simulink model "sim_BTMS"  (R2018b)
settings: Solver=FixedStepAuto  StartTime=0.0  StopTime=SimPara.t_sim  FixedStep=SimPara.t_step  RelTol=1e-3
values from neighbouring files (symbols this model uses):
  p = epe(jj).p    [main_sim_BTMS.m]    (also in main_sim_BTMS_1_system_setup.m = epe_mod(jj).p)
  SysPara = rmfield(SysPara, {'p','s'})    [main_sim_BTMS_1_system_setup.m]
undefined symbols (not defined in the file or in its folder): A, BatPara, BTMSConfig, i, LSAPara, SimPara, x2_cal, x3_cal, x_cal
libraries: simulink x14, dspstat3 x7, dspindex x1
(part 2 of 4)

== system sim_BTMS/Battery system simulation/Static and dynamic LIB parameters/LIB Parameter Look-Ups ==
  note: Determination of the current BatPara cell parameter set, dependent on SOC, C-Rate and Temperature of every individual cell of the battery system.
  note: RC-Element 1
  note: RC-Element 2
  note: RC-Element 3
  note: RC-Element 4
  BatState_th_in : Inport
  BatState_el_in : Inport  Port=2
  Apply Deviation Map to C_A : Constant  Value=BatPara.electrical.C_A*SysPara.DeviationMap.C_A  VectorParams1D=off
  Bus Creator : BusCreator  Inputs=10
  Bus Selector : BusSelector  OutputSignals=SOC,I_cell [A]
  Bus Selector1 : BusSelector  OutputSignals=T_cell [°C]
  Divide : Product  Inputs=*/
  Lookup C1 : Lookup_n-D  NumberOfTableDimensions=3  BreakpointsForDimension1=BatPara.electrical.dyn.SOC  BreakpointsForDimension2=BatPara.electrical.dyn.T  BreakpointsForDimension3=BatPara.electrical.dyn.C_rate  BeginIndexSearchUsingPreviousIndexResult=on  Table=BatPara.electrical.dyn.C1  ExtrapMethod=Clip  RemoveProtectionInput=on  UseLastTableValue=on  InternalRulePriority=Speed  RndMeth=Simplest  InputSameDT=on
  Lookup C2 : Lookup_n-D  NumberOfTableDimensions=3  BreakpointsForDimension1=BatPara.electrical.dyn.SOC  BreakpointsForDimension2=BatPara.electrical.dyn.T  BreakpointsForDimension3=BatPara.electrical.dyn.C_rate  BeginIndexSearchUsingPreviousIndexResult=on  Table=BatPara.electrical.dyn.C2  ExtrapMethod=Clip  RemoveProtectionInput=on  UseLastTableValue=on  InternalRulePriority=Speed  RndMeth=Simplest  InputSameDT=on
  Lookup C3 : Lookup_n-D  NumberOfTableDimensions=3  BreakpointsForDimension1=BatPara.electrical.dyn.SOC  BreakpointsForDimension2=BatPara.electrical.dyn.T  BreakpointsForDimension3=BatPara.electrical.dyn.C_rate  BeginIndexSearchUsingPreviousIndexResult=on  Table=BatPara.electrical.dyn.C3  ExtrapMethod=Clip  RemoveProtectionInput=on  UseLastTableValue=on  InternalRulePriority=Speed  RndMeth=Simplest  InputSameDT=on
  Lookup C4 : Lookup_n-D  NumberOfTableDimensions=3  BreakpointsForDimension1=BatPara.electrical.dyn.SOC  BreakpointsForDimension2=BatPara.electrical.dyn.T  BreakpointsForDimension3=BatPara.electrical.dyn.C_rate  BeginIndexSearchUsingPreviousIndexResult=on  Table=BatPara.electrical.dyn.C4  ExtrapMethod=Clip  RemoveProtectionInput=on  UseLastTableValue=on  InternalRulePriority=Speed  RndMeth=Simplest  InputSameDT=on
  Lookup R1 : Lookup_n-D  NumberOfTableDimensions=3  BreakpointsForDimension1=BatPara.electrical.dyn.SOC  BreakpointsForDimension2=BatPara.electrical.dyn.T  BreakpointsForDimension3=BatPara.electrical.dyn.C_rate  BeginIndexSearchUsingPreviousIndexResult=on  Table=BatPara.electrical.dyn.R1  ExtrapMethod=Clip  RemoveProtectionInput=on  UseLastTableValue=on  InternalRulePriority=Speed  RndMeth=Simplest  InputSameDT=on
  Lookup R2 : Lookup_n-D  NumberOfTableDimensions=3  BreakpointsForDimension1=BatPara.electrical.dyn.SOC  BreakpointsForDimension2=BatPara.electrical.dyn.T  BreakpointsForDimension3=BatPara.electrical.dyn.C_rate  BeginIndexSearchUsingPreviousIndexResult=on  Table=BatPara.electrical.dyn.R2  ExtrapMethod=Clip  RemoveProtectionInput=on  UseLastTableValue=on  InternalRulePriority=Speed  RndMeth=Simplest  InputSameDT=on
  Lookup R3 : Lookup_n-D  NumberOfTableDimensions=3  BreakpointsForDimension1=BatPara.electrical.dyn.SOC  BreakpointsForDimension2=BatPara.electrical.dyn.T  BreakpointsForDimension3=BatPara.electrical.dyn.C_rate  BeginIndexSearchUsingPreviousIndexResult=on  Table=BatPara.electrical.dyn.R3  ExtrapMethod=Clip  RemoveProtectionInput=on  UseLastTableValue=on  InternalRulePriority=Speed  RndMeth=Simplest  InputSameDT=on
  Lookup R4 : Lookup_n-D  NumberOfTableDimensions=3  BreakpointsForDimension1=BatPara.electrical.dyn.SOC  BreakpointsForDimension2=BatPara.electrical.dyn.T  BreakpointsForDimension3=BatPara.electrical.dyn.C_rate  BeginIndexSearchUsingPreviousIndexResult=on  Table=BatPara.electrical.dyn.R4  ExtrapMethod=Clip  RemoveProtectionInput=on  UseLastTableValue=on  InternalRulePriority=Speed  RndMeth=Simplest  InputSameDT=on
  Lookup R_0 : Lookup_n-D  NumberOfTableDimensions=3  BreakpointsForDimension1=BatPara.electrical.dyn.SOC  BreakpointsForDimension2=BatPara.electrical.dyn.T  BreakpointsForDimension3=BatPara.electrical.dyn.C_rate  BeginIndexSearchUsingPreviousIndexResult=on  Table=BatPara.electrical.dyn.R_0  ExtrapMethod=Clip  RemoveProtectionInput=on  UseLastTableValue=on  InternalRulePriority=Speed  RndMeth=Simplest  InputSameDT=on
  BatPara_el_uniform : Outport
  wires:
  Bus Selector/1 -> Lookup R_0/1, Lookup R1/1, Lookup C1/1, Lookup C4/1, Lookup R4/1, Lookup C3/1, Lookup R3/1, Lookup C2/1, Lookup R2/1  "<SOC>"
  Divide/1 -> Lookup R_0/2, Lookup R1/2, Lookup C1/2, Lookup C4/2, Lookup R4/2, Lookup C3/2, Lookup R3/2, Lookup C2/2, Lookup R2/2
  Lookup R_0/1 -> Bus Creator/1  "R_0 [Ohm]"
  Bus Selector1/1 -> Lookup R3/3, Lookup C3/3, Lookup R4/3, Lookup C4/3, Lookup R_0/3, Lookup R1/3, Lookup C1/3, Lookup R2/3, Lookup C2/3  "<T_cell [°C]>"
  Lookup R1/1 -> Bus Creator/2  "R1 [Ohm]"
  Lookup R2/1 -> Bus Creator/4  "R2 [Ohm]"
  Lookup C1/1 -> Bus Creator/3  "C1 [F]"
  Lookup C2/1 -> Bus Creator/5  "C2 [F]"
  BatState_el_in/1 -> Bus Selector/1
  Apply Deviation Map to C_A/1 -> Divide/2, Bus Creator/10  "C_A [Ah]"
  Bus Creator/1 -> BatPara_el_uniform/1
  Bus Selector/2 -> Divide/1  "<I_cell [A]>"
  BatState_th_in/1 -> Bus Selector1/1
  Lookup C4/1 -> Bus Creator/9  "C4 [F]"
  Lookup C3/1 -> Bus Creator/7  "C3 [F]"
  Lookup R4/1 -> Bus Creator/8  "R4 [Ohm]"
  Lookup R3/1 -> Bus Creator/6  "R3 [Ohm]"

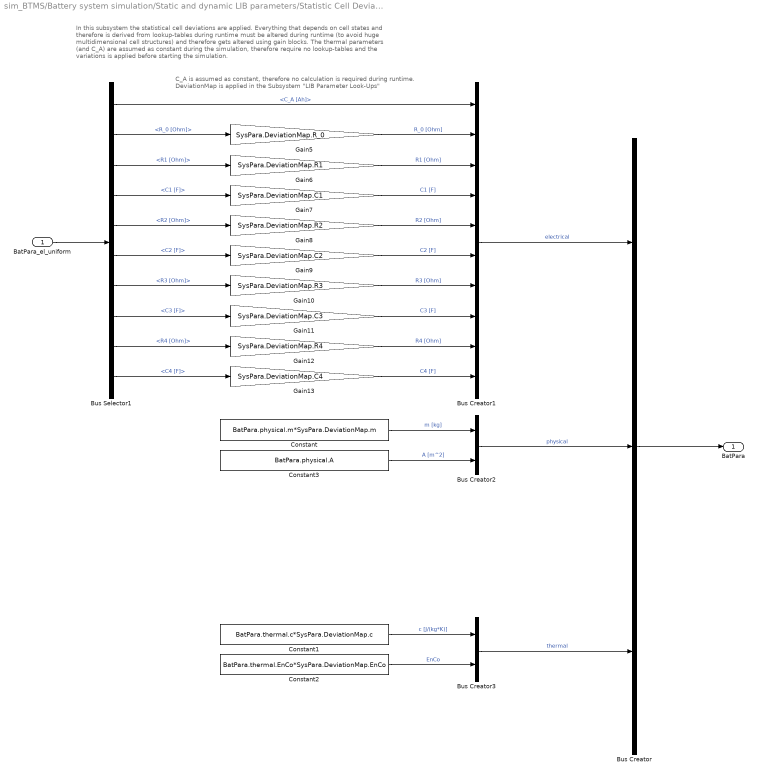
== system sim_BTMS/Battery system simulation/Static and dynamic LIB parameters/Statistic Cell Deviations ==
  note: In this subsystem the statistical cell deviations are applied. Everything that depends on cell states and therefore is derived from lookup-tables during runtime
      | must be altered during runtime (to avoid huge multidimensional cell structures) and therefore gets altered using gain blocks. The thermal parameters (and C_A)
      | are assumed as constant during the simulation, therefore require no lookup-tables and the variations is applied before starting the simulation.
  note: C_A is assumed as constant, therefore no calculation is required during runtime.
      | DeviationMap is applied in the Subsystem "LIB Parameter Look-Ups"
  "BatPara_el_uniform " : Inport
  Bus Creator : BusCreator  Inputs=3
  Bus Creator1 : BusCreator  Inputs=10
  Bus Creator2 : BusCreator  Inputs=2
  Bus Creator3 : BusCreator  Inputs=2
  Bus Selector1 : BusSelector  OutputSignals=C_A [Ah],R_0 [Ohm],R1 [Ohm],C1 [F],R2 [Ohm],C2 [F],R3 [Ohm],C3 [F],R4 [Ohm],C4 [F]
  Constant : Constant  Value=BatPara.physical.m*SysPara.DeviationMap.m
  Constant1 : Constant  Value=BatPara.thermal.c*SysPara.DeviationMap.c
  Constant2 : Constant  Value=BatPara.thermal.EnCo*SysPara.DeviationMap.EnCo
  Constant3 : Constant  Value=BatPara.physical.A
  Gain10 : Gain  Gain=SysPara.DeviationMap.R3
  Gain11 : Gain  Gain=SysPara.DeviationMap.C3
  Gain12 : Gain  Gain=SysPara.DeviationMap.R4
  Gain13 : Gain  Gain=SysPara.DeviationMap.C4
  Gain5 : Gain  Gain=SysPara.DeviationMap.R_0
  Gain6 : Gain  Gain=SysPara.DeviationMap.R1
  Gain7 : Gain  Gain=SysPara.DeviationMap.C1
  Gain8 : Gain  Gain=SysPara.DeviationMap.R2
  Gain9 : Gain  Gain=SysPara.DeviationMap.C2
  BatPara : Outport
  wires:
  "BatPara_el_uniform "/1 -> Bus Selector1/1
  Bus Selector1/2 -> Gain5/1  "<R_0 [Ohm]>"
  Bus Selector1/3 -> Gain6/1  "<R1 [Ohm]>"
  Bus Selector1/4 -> Gain7/1  "<C1 [F]>"
  Bus Selector1/5 -> Gain8/1  "<R2 [Ohm]>"
  Bus Selector1/6 -> Gain9/1  "<C2 [F]>"
  Bus Selector1/7 -> Gain10/1  "<R3 [Ohm]>"
  Bus Selector1/8 -> Gain11/1  "<C3 [F]>"
  Bus Selector1/9 -> Gain12/1  "<R4 [Ohm]>"
  Bus Selector1/10 -> Gain13/1  "<C4 [F]>"
  Bus Selector1/1 -> Bus Creator1/1  "<C_A [Ah]>"
  Gain5/1 -> Bus Creator1/2  "R_0 [Ohm]"
  Gain6/1 -> Bus Creator1/3  "R1 [Ohm]"
  Gain7/1 -> Bus Creator1/4  "C1 [F]"
  Gain8/1 -> Bus Creator1/5  "R2 [Ohm]"
  Gain9/1 -> Bus Creator1/6  "C2 [F]"
  Gain10/1 -> Bus Creator1/7  "R3 [Ohm]"
  Gain11/1 -> Bus Creator1/8  "C3 [F]"
  Gain12/1 -> Bus Creator1/9  "R4 [Ohm]"
  Gain13/1 -> Bus Creator1/10  "C4 [F]"
  Bus Creator1/1 -> Bus Creator/1  "electrical"
  Bus Creator2/1 -> Bus Creator/2  "physical"
  Constant/1 -> Bus Creator2/1  "m [kg]"
  Constant1/1 -> Bus Creator3/1  "c [J/(kg*K)]"
  Constant2/1 -> Bus Creator3/2  "EnCo"
  Constant3/1 -> Bus Creator2/2  "A [m^2]"
  Bus Creator/1 -> BatPara/1
  Bus Creator3/1 -> Bus Creator/3  "thermal"

== system sim_BTMS/Battery system simulation/Thermal Submodel/Cell heat transport and heat dissipation ==
  PQ_cell : Inport
  BatPara : Inport  Port=2
  T_cell_in : Inport  Port=3
  alpha_cell_ambient : Inport  Port=4
  T_cell_ambient : Inport  Port=5
  Enable : EnablePort
  Heat dissipation model : Subsystem
  Heat transfer between cells : Subsystem  Variant=on
  Lumped mass thermal cell model : Subsystem  VariantControl=SimPara.heat_exchange_enable == 0
  T_cell [°C] : Outport  InitialOutput=SysPara.BatStateInit.thermal.T_cell
  PQ_ambient [W] : Outport  Port=2  InitialOutput=0
  PQ_transfer [W] : Outport  Port=3  InitialOutput=0
  wires:
  Lumped mass thermal cell model/1(T_cell [°C]) -> T_cell [°C]/1
  PQ_cell/1 -> Lumped mass thermal cell model/1(PQ_cell)
  BatPara/1 -> Heat dissipation model/2(BatPara), Lumped mass thermal cell model/2(BatPara)
  T_cell_in/1 -> Heat transfer between cells/1(T_cell_in), Heat dissipation model/1(T_cells_in), Lumped mass thermal cell model/3(T_cell_in)
  T_cell_ambient/1 -> Heat dissipation model/3(T_cell_ambient)
  alpha_cell_ambient/1 -> Heat dissipation model/4(alpha_cell_ambient)
  Heat dissipation model/1(PQ_ambient) -> PQ_ambient [W]/1, Lumped mass thermal cell model/4(PQ_ambient)
  Heat transfer between cells/1(PQ_transfer) -> PQ_transfer [W]/1, Lumped mass thermal cell model/5(PQ_transfer)

== system sim_BTMS/Battery system simulation/Thermal Submodel/Irreversible heat generation ==
  note: Calculation of ohmic/irreversible heat losses:
      |
      | -> Equation PQ_Cells,irr = R_Cells,total * I_Cells^2
      | -> R_Cells is the sum of all voltage drops in the cell (internal resistance and RC-Elements)
  U_R [V] : Inport
  U_RC : Inport  Port=2
  I_Cells [A] : Inport  Port=3
  Abs : Abs
  Add : Sum
  Bus Selector : BusSelector  OutputSignals=sum_U_RC [V]
  Product : Product  Inputs=**  RndMeth=Zero
  PQ_cell,irr [W] : Outport
  wires:
  I_Cells [A]/1 -> Product/2
  Add/1 -> Product/1
  Product/1 -> Abs/1
  U_R [V]/1 -> Add/1
  U_RC/1 -> Bus Selector/1
  Abs/1 -> PQ_cell,irr [W]/1  "PQ_cell,irr"
  Bus Selector/1 -> Add/2  "<sum_U_RC [V]>"

== system sim_BTMS/Battery system simulation/Thermal Submodel/Reversible heat generation ==
  note: Calculation of reversible heat losses in the cells
      |
      | PQ_Cells,rev = - I_cell * T_cell * (dUocv/dT_cell) = - I_cell * T_cell * EnCo
      |
      | Eddahech et al., 2013 - Thermal characterization of a high-power lithium-ion battery
  I_Cells [A] : Inport
  T_Cells [°C] : Inport  Port=2
  BatPara : Inport  Port=3
  Bus Selector : BusSelector  OutputSignals=thermal.EnCo
  Gain : Gain  Gain=-1
  Product : Product  Inputs=***  RndMeth=Zero
  PQ_cell,rev [W] : Outport
  wires:
  BatPara/1 -> Bus Selector/1
  Product/1 -> Gain/1
  T_Cells [°C]/1 -> Product/3
  I_Cells [A]/1 -> Product/1
  Gain/1 -> PQ_cell,rev [W]/1  "PQ_cell,rev"
  Bus Selector/1 -> Product/2  "<EnCo>"

== system sim_BTMS/Monitoring and Logging/Load Spectrum Analysis/Load Spectrum Analysis OFF ==
  BatState_el : Inport
  BatState_th : Inport  Port=2
  BatPara : Inport  Port=3
  Terminator : Terminator
  Terminator1 : Terminator
  Terminator2 : Terminator
  wires:
  BatState_el/1 -> Terminator/1
  BatState_th/1 -> Terminator1/1
  BatPara/1 -> Terminator2/1

== system sim_BTMS/Monitoring and Logging/Load Spectrum Analysis/Load Spectrum Analysis ON ==
  BatState_el : Inport
  BatState_th : Inport  Port=2
  BatPara : Inport  Port=3
  Bus Selector : BusSelector  OutputSignals=SOC,I_cell [A],U_cell [V]
  Bus Selector1 : BusSelector  OutputSignals=T_cell [°C]
  Bus Selector2 : BusSelector  OutputSignals=electrical.C_A [Ah]
  Load Spectrum Analysis ON : Subsystem  VariantControl=SimPara.LoadSpectra == 1
  wires:
  BatState_el/1 -> Bus Selector/1
  BatState_th/1 -> Bus Selector1/1
  BatPara/1 -> Bus Selector2/1
  Bus Selector/1 -> Load Spectrum Analysis ON/1(SOC)  "<SOC>"
  Bus Selector/2 -> Load Spectrum Analysis ON/2(I_cell [A])  "<I_cell [A]>"
  Bus Selector/3 -> Load Spectrum Analysis ON/3(U_Cell [A])  "<U_cell [V]>"
  Bus Selector1/1 -> Load Spectrum Analysis ON/4(T_cell [°C])  "<T_cell [°C]>"
  Bus Selector2/1 -> Load Spectrum Analysis ON/5(C_A [Ah])  "<C_A [Ah]>"

== system sim_BTMS/Monitoring and Logging/Logging of Variables/Calc Temp Gradient ==
  T_cell : Inport
  Abs : Abs
  Add : Sum  Inputs=-+
  MinMax : MinMax
  MinMax1 : MinMax  Function=max
  Reshape : Reshape
  T_cell_gradient : Outport
  wires:
  T_cell/1 -> Reshape/1
  MinMax/1 -> Add/1
  MinMax1/1 -> Add/2
  Add/1 -> Abs/1
  Abs/1 -> T_cell_gradient/1
  Reshape/1 -> MinMax1/1, MinMax/1

== system sim_BTMS/Monitoring and Logging/Temperature Sensor Simulation/Enable//disable temperature sensors ==
  T_cell : Inport
  TempSensors OFF : Subsystem  VariantControl=SimPara.TempSensors_enable==0
  TempSensors ON : Subsystem  VariantControl=SimPara.TempSensors_enable==1
  T_sensors [°C] : Outport

== system sim_BTMS/Monitoring and Logging/Temperature Sensor Simulation/Rebuild bus structure ==
  T_sensors : Inport
  Bat_state_th_in : Inport  Port=2
  Bus Creator1 : BusCreator  Inputs=7
  Bus Selector1 : BusSelector  OutputSignals=PQ_cell [W],T_cell [°C],T_cell_ambient,alpha_cell_ambient,PQ_ambient [W],PQ_transfer [W]
  bat_state_th_out : Outport
  wires:
  Bus Selector1/4 -> Bus Creator1/4  "<alpha_cell_ambient>"
  Bus Selector1/1 -> Bus Creator1/1  "<PQ_cell [W]>"
  Bus Selector1/2 -> Bus Creator1/2  "<T_cell [°C]>"
  T_sensors/1 -> Bus Creator1/7
  Bus Selector1/3 -> Bus Creator1/3  "<T_cell_ambient>"
  Bat_state_th_in/1 -> Bus Selector1/1
  Bus Creator1/1 -> bat_state_th_out/1  "bat_state_th"
  Bus Selector1/5 -> Bus Creator1/5  "<PQ_ambient [W]>"
  Bus Selector1/6 -> Bus Creator1/6  "<PQ_transfer [W]>"

== system sim_BTMS/Battery system simulation/Electrical Submodel/Electric potential (single cell)/Cell ECM RC-element 1 ==
  BatState_In : Inport
  BatPara : Inport  Port=2
  dt [s] : Inport  Port=3
  Enable : EnablePort
  Bus Selector : BusSelector  OutputSignals=U_RC.U_RC1 [V],I_cell [A]
  Bus Selector1 : BusSelector  OutputSignals=electrical.R1 [Ohm],electrical.C1 [F]
  Constant : Constant  VectorParams1D=off
  Gain : Gain  Gain=-1
  Math Function : Math  SaturateOnIntegerOverflow=on
  Product : Product  Inputs=**  RndMeth=Zero
  Product1 : Product  Inputs=/*  RndMeth=Zero
  Product2 : Product  Inputs=***  RndMeth=Zero
  Product3 : Product  Inputs=**  RndMeth=Zero
  Sum : Sum  Inputs=-+
  Sum1 : Sum
  U_RC1 [V] : Outport  OutputWhenDisabled=reset  InitialOutput=zeros(SysPara.p,SysPara.s)
  wires:
  Product/1 -> Product1/1
  Product3/1 -> Sum1/1
  Product1/1 -> Gain/1
  Sum1/1 -> U_RC1 [V]/1
  Gain/1 -> Math Function/1
  Product2/1 -> Sum1/2
  Bus Selector/1 -> Product3/1  "<U_RC1 [V]>"
  Math Function/1 -> Sum/1, Product3/2
  Sum/1 -> Product2/1
  Bus Selector1/1 -> Product2/2, Product/1  "<R1 [Ohm]>"
  BatPara/1 -> Bus Selector1/1
  dt [s]/1 -> Product1/2
  Bus Selector/2 -> Product2/3  "<I_cell [A]>"
  BatState_In/1 -> Bus Selector/1
  Bus Selector1/2 -> Product/2  "<C1 [F]>"
  Constant/1 -> Sum/2

== system sim_BTMS/Battery system simulation/Electrical Submodel/Electric potential (single cell)/Cell ECM RC-element 2 ==
  BatState_In : Inport
  BatPara : Inport  Port=2
  dt [s] : Inport  Port=3
  Enable : EnablePort
  Bus Selector : BusSelector  OutputSignals=U_RC.U_RC2 [V],I_cell [A]
  Bus Selector1 : BusSelector  OutputSignals=electrical.R2 [Ohm],electrical.C2 [F]
  Constant : Constant  VectorParams1D=off
  Gain : Gain  Gain=-1
  Math Function : Math  SaturateOnIntegerOverflow=on
  Product : Product  Inputs=**  RndMeth=Zero
  Product1 : Product  Inputs=/*  RndMeth=Zero
  Product2 : Product  Inputs=***  RndMeth=Zero
  Product3 : Product  Inputs=**  RndMeth=Zero
  Sum : Sum  Inputs=-+
  Sum1 : Sum
  U_RC2 [V] : Outport  OutputWhenDisabled=reset  InitialOutput=zeros(SysPara.p,SysPara.s)
  wires:
  Product/1 -> Product1/1
  Product3/1 -> Sum1/1
  Product1/1 -> Gain/1
  Sum1/1 -> U_RC2 [V]/1
  Gain/1 -> Math Function/1
  Product2/1 -> Sum1/2
  Bus Selector/1 -> Product3/1  "<U_RC2 [V]>"
  Math Function/1 -> Sum/1, Product3/2
  Sum/1 -> Product2/1
  Bus Selector1/1 -> Product2/2, Product/1  "<R2 [Ohm]>"
  BatPara/1 -> Bus Selector1/1
  dt [s]/1 -> Product1/2
  Bus Selector/2 -> Product2/3  "<I_cell [A]>"
  BatState_In/1 -> Bus Selector/1
  Bus Selector1/2 -> Product/2  "<C2 [F]>"
  Constant/1 -> Sum/2

== system sim_BTMS/Battery system simulation/Electrical Submodel/Electric potential (single cell)/Cell ECM RC-element 3 ==
  BatState_In : Inport
  BatPara : Inport  Port=2
  dt [s] : Inport  Port=3
  Enable : EnablePort
  Bus Selector : BusSelector  OutputSignals=U_RC.U_RC3 [V],I_cell [A]
  Bus Selector1 : BusSelector  OutputSignals=electrical.R3 [Ohm],electrical.C3 [F]
  Constant : Constant  VectorParams1D=off
  Gain : Gain  Gain=-1
  Math Function : Math  SaturateOnIntegerOverflow=on
  Product : Product  Inputs=**  RndMeth=Zero
  Product1 : Product  Inputs=/*  RndMeth=Zero
  Product2 : Product  Inputs=***  RndMeth=Zero
  Product3 : Product  Inputs=**  RndMeth=Zero
  Sum : Sum  Inputs=-+
  Sum1 : Sum
  U_RC3 [V] : Outport  OutputWhenDisabled=reset  InitialOutput=zeros(SysPara.p,SysPara.s)
  wires:
  Product/1 -> Product1/1
  Product3/1 -> Sum1/1
  Product1/1 -> Gain/1
  Sum1/1 -> U_RC3 [V]/1
  Gain/1 -> Math Function/1
  Product2/1 -> Sum1/2
  Bus Selector/1 -> Product3/1  "<U_RC3 [V]>"
  Math Function/1 -> Sum/1, Product3/2
  Sum/1 -> Product2/1
  Bus Selector1/1 -> Product2/2, Product/1  "<R3 [Ohm]>"
  BatPara/1 -> Bus Selector1/1
  dt [s]/1 -> Product1/2
  Bus Selector/2 -> Product2/3  "<I_cell [A]>"
  BatState_In/1 -> Bus Selector/1
  Bus Selector1/2 -> Product/2  "<C3 [F]>"
  Constant/1 -> Sum/2

== system sim_BTMS/Battery system simulation/Electrical Submodel/Electric potential (single cell)/Cell ECM RC-element 4 ==
  BatState_In : Inport
  BatPara : Inport  Port=2
  dt [s] : Inport  Port=3
  Enable : EnablePort
  Bus Selector : BusSelector  OutputSignals=U_RC.U_RC4 [V],I_cell [A]
  Bus Selector1 : BusSelector  OutputSignals=electrical.R4 [Ohm],electrical.C4 [F]
  Constant : Constant  VectorParams1D=off
  Gain : Gain  Gain=-1
  Math Function : Math  SaturateOnIntegerOverflow=on
  Product : Product  Inputs=**  RndMeth=Zero
  Product1 : Product  Inputs=/*  RndMeth=Zero
  Product2 : Product  Inputs=***  RndMeth=Zero
  Product3 : Product  Inputs=**  RndMeth=Zero
  Sum : Sum  Inputs=-+
  Sum1 : Sum
  U_RC4 [V] : Outport  OutputWhenDisabled=reset  InitialOutput=zeros(SysPara.p,SysPara.s)
  wires:
  Product/1 -> Product1/1
  Product3/1 -> Sum1/1
  Product1/1 -> Gain/1
  Sum1/1 -> U_RC4 [V]/1
  Gain/1 -> Math Function/1
  Product2/1 -> Sum1/2
  Bus Selector/1 -> Product3/1  "<U_RC4 [V]>"
  Math Function/1 -> Sum/1, Product3/2
  Sum/1 -> Product2/1
  Bus Selector1/1 -> Product2/2, Product/1  "<R4 [Ohm]>"
  BatPara/1 -> Bus Selector1/1
  dt [s]/1 -> Product1/2
  Bus Selector/2 -> Product2/3  "<I_cell [A]>"
  BatState_In/1 -> Bus Selector/1
  Bus Selector1/2 -> Product/2  "<C4 [F]>"
  Constant/1 -> Sum/2

== system sim_BTMS/Battery system simulation/Electrical Submodel/Electric potential (single cell)/Cell Hysteresis Voltage ==
  note: Zugrunde liegende Formel aus "Verbrugge, 2007 - Adaptive, multi-parameter battery state estimator with optimized time weighting factors"
  note: Wenn kein Hysteresemodell verwendet werden soll
      |  beta = 0 setzen
  BatState_In : Inport
  dt [s] : Inport  Port=2
  Add : Sum  Inputs=-+
  Add1 : Sum
  Bus Selector : BusSelector  OutputSignals=U_Hysteresis [V],I_cell [A],SOC
  Product : Product
  Product1 : Product  Inputs=4
  Sign : Signum
  V_H,max(SOC) : Lookup_n-D  NumberOfTableDimensions=1  BreakpointsForDimension1=BatPara.electrical.OCV.SOC  BeginIndexSearchUsingPreviousIndexResult=on  Table=BatPara.electrical.OCV.U_hyst  ExtrapMethod=Clip  DiagnosticForOutOfRangeInput=Warning  RemoveProtectionInput=on  UseLastTableValue=on  InternalRulePriority=Speed  RndMeth=Simplest  InputSameDT=on
  beta : Constant  Value=BatPara.electrical.OCV.beta_hyst  VectorParams1D=off
  U_Hysteresis [V] : Outport
  wires:
  Bus Selector/2 -> Sign/1, Product1/3  "<I_cell [A]>"
  Bus Selector/3 -> V_H,max(SOC)/1  "<SOC>"
  V_H,max(SOC)/1 -> Add/2
  Add/1 -> Product1/4  "V_H,max-sign(I)*V_H"
  dt [s]/1 -> Product1/2
  Product1/1 -> Add1/2
  Add1/1 -> U_Hysteresis [V]/1
  Sign/1 -> Product/2  "sign(I)"
  Product/1 -> Add/1
  BatState_In/1 -> Bus Selector/1
  Bus Selector/1 -> Add1/1, Product/1  "<U_Hysteresis [V]>"
  beta/1 -> Product1/1

== system sim_BTMS/Battery system simulation/Electrical Submodel/Electric potential (single cell)/Cell Open-Circuit-Voltage ==
  SOC [-] : Inport
  BatPara : Inport  Port=2
  SOC --> U : Lookup_n-D  NumberOfTableDimensions=1  BreakpointsForDimension1=BatPara.electrical.OCV.SOC  BreakpointsForDimension2=[1:3]  IndexSearchMethod=Linear search  BeginIndexSearchUsingPreviousIndexResult=on  Table=BatPara.electrical.OCV.U  DiagnosticForOutOfRangeInput=Warning  RemoveProtectionInput=on  RndMeth=Simplest  InputSameDT=on
  Terminator : Terminator
  U_OCV [V] : Outport
  wires:
  SOC [-]/1 -> SOC --> U/1
  SOC --> U/1 -> U_OCV [V]/1
  BatPara/1 -> Terminator/1

== system sim_BTMS/Battery system simulation/Electrical Submodel/Electric potential (single cell)/Cell SOC ==
  BatPara : Inport
  BatState_In : Inport  Port=2
  dt [s] : Inport  Port=3
  Ah in As : Gain  Gain=3600
  Bus Selector : BusSelector  OutputSignals=electrical.C_A [Ah]
  Bus Selector1 : BusSelector  OutputSignals=I_cell [A],SOC
  Product : Product  Inputs=**/  RndMeth=Zero
  Sum : Sum
  SOC [-] : Outport
  wires:
  Bus Selector1/2 -> Sum/2  "<SOC>"
  Product/1 -> Sum/1  "delta_SOC"
  Bus Selector/1 -> Ah in As/1  "<C_A [Ah]>"
  Ah in As/1 -> Product/3
  Bus Selector1/1 -> Product/2  "<I_cell [A]>"
  dt [s]/1 -> Product/1
  BatState_In/1 -> Bus Selector1/1
  BatPara/1 -> Bus Selector/1
  Sum/1 -> SOC [-]/1

== system sim_BTMS/Battery system simulation/Thermal Submodel/Cell heat transport and heat dissipation/Heat dissipation model ==
  note: Determination of the heat fluxes between the cells and their environments:
      | à No heat exchange between adjacent cells in the battery pack (optionally done in subsystem 'Heat transfer between cells')
      | à Each individual cell is independently viewed and has its own environmental temperature and heat transfer coefficient to the environment (defined by model input 'BTMS_input' at the top level of the model).
      | à Heat flow between a cell and its environment only via convection
      | PQ_Ambient* = alpha_cell_mbient * A * (T_cell_ambient - T_cell*)
  T_cells_in : Inport
  BatPara : Inport  Port=2
  T_cell_ambient : Inport  Port=3
  alpha_cell_ambient : Inport  Port=4
  Bus Selector2 : BusSelector  OutputSignals=physical.A [m^2]
  Product : Product  Inputs=3
  Subtract : Sum  Inputs=+-
  PQ_ambient : Outport
  wires:
  Bus Selector2/1 -> Product/2  "<A [m^2]>"
  T_cells_in/1 -> Subtract/2
  Subtract/1 -> Product/3
  BatPara/1 -> Bus Selector2/1
  T_cell_ambient/1 -> Subtract/1
  Product/1 -> PQ_ambient/1  "PQ_ambient [W]"
  alpha_cell_ambient/1 -> Product/1

== system sim_BTMS/Battery system simulation/Thermal Submodel/Cell heat transport and heat dissipation/Heat transfer between cells ==
  note: Variants:
      |
      | - Heat transfer model switched OFF: No heat transfer between cells, PQ_transfer is always 0
      |
      | - Heat transfer model switched OFF: Heat transfer between cells is simulated and a heat flux from/to every cell is computed.
  T_cell_in : Inport
  Heat transfer model switched OFF : Subsystem  VariantControl=SimPara.heat_exchange_enable == 0
  Heat transfer model switched ON : Subsystem  VariantControl=SimPara.heat_exchange_enable == 1
  PQ_transfer : Outport  InitialOutput=SysPara.BatStateInit.thermal.T_cell

== system sim_BTMS/Battery system simulation/Thermal Submodel/Cell heat transport and heat dissipation/Lumped mass thermal cell model ==
  note: Determination of the heat outputs which allow a temperature change of the cells:
      | à Sum of the individual heat outputs or flows for each cell
      | à The "Unit Delay" allows the heat outputs of the cells to be viewed from the previous evaluation time.
      | à By subtracting the temperatures of the cells from their ambient temperatures, the heat flows between the cells and their environments are properly defined for the equation
      | PQ_Temperature = PQ_cells + PQ_ambient + PQ_transfer
  note: Determination of the quantities of heat that allow the temperature of the cells to change:
      | à Heat quantity is integral of the heat output over time.
      | à Assumption that the heat outputs, which enable a temperature change of the cells, remain constant from the previous evaluation time until the current evaluation time.
      | à dt is time difference between two evaluations
      | Q_Temperature = PQ_Temperature* * dt
  note: Determination of the cell temperatures at the current evaluation time:
      | à Q_Temperature result in current temperature changes of the cells compared to the previous evaluation time.
      | Q_Temperature = m * c * (T_cell - T_cell*)
      | à T_cell = Q_Temperature / (m * c) + T_cell*
  PQ_cell : Inport
  BatPara : Inport  Port=2
  T_cell_in : Inport  Port=3
  PQ_ambient : Inport  Port=4
  PQ_transfer : Inport  Port=5
  Add1 : Sum
  Bus Selector1 : BusSelector  OutputSignals=physical.m [kg],thermal.c [J/(kg*K)]
  Divide : Product  Inputs=*/
  Product1 : Product
  Product2 : Product
  Subtract1 : Sum  Inputs=+++
  dt : Subsystem
  T_cell [°C] : Outport
  wires:
  T_cell_in/1 -> Add1/2
  BatPara/1 -> Bus Selector1/1
  PQ_cell/1 -> Subtract1/1
  Bus Selector1/1 -> Product2/1  "<m [kg]>"
  Bus Selector1/2 -> Product2/2  "<c [J/(kg*K)]>"
  Subtract1/1 -> Product1/2  "PQ_Temperature"
  dt/1(dt [s]) -> Product1/1
  Divide/1 -> Add1/1
  Product2/1 -> Divide/2
  Add1/1 -> T_cell [°C]/1  "T_cell [°C]"
  Product1/1 -> Divide/1  "Q_Temperature"
  PQ_ambient/1 -> Subtract1/2
  PQ_transfer/1 -> Subtract1/3
